simulink model "ds_adc_system"  (R2021b)
settings: Solver=VariableStepAuto  StartTime=0.0  StopTime=1 - 1/5.12e6  RelTol=1e-3
undefined symbols (not defined in the file): a1, a2, b1, b2, c1, c2, DiscIntNeverNeededParam, f, vin
libraries: simulink_extras x2, dspsigops x1
settings Model: Creator=Raymond.Yang  LastModifiedBy=Raymond.Yang
settings SolverCC: AlgebraicLoopSolver=TrustRegion
settings DebuggingCC: SFMachineParentedDataDiag=warning

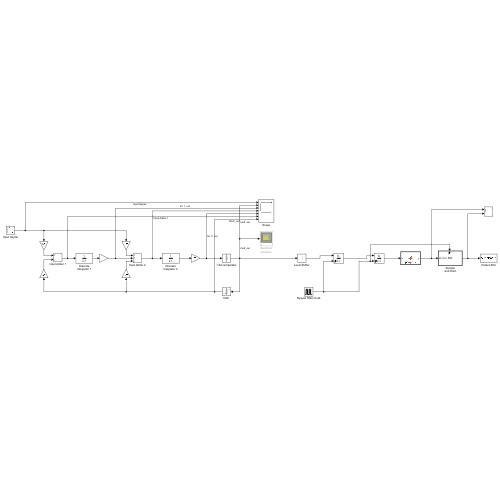
[thumbnail: Simulink's stored preview of the top-level diagram]
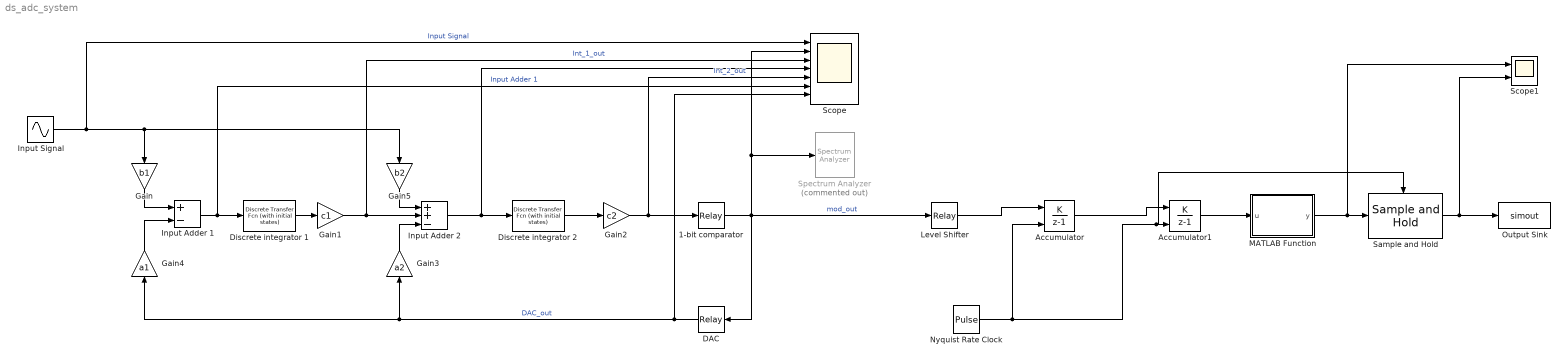
== system ds_adc_system ==
  1-bit comparator : Relay  OnSwitchValue=0  OffSwitchValue=0  OffOutputValue=-1
  Accumulator : DiscreteIntegrator  IntegratorMethod=Accumulation: Forward Euler  ExternalReset=rising  SampleTime=-1  ICPrevOutput=DiscIntNeverNeededParam  ICPrevScaledInput=DiscIntNeverNeededParam
  Accumulator1 : DiscreteIntegrator  IntegratorMethod=Accumulation: Forward Euler  ExternalReset=rising  SampleTime=-1  ICPrevOutput=DiscIntNeverNeededParam  ICPrevScaledInput=DiscIntNeverNeededParam
  DAC : Relay  OnSwitchValue=1  OffSwitchValue=-1  OnOutputValue=0.9  OffOutputValue=-0.9
  Discrete integrator 1 : simulink_extras/Additional Discrete/Discrete Transfer Fcn (with initial states)  N=[1]  D="[1  -1]"  X0=0  TS=-1
      settings: SourceProductBaseCode=SL
  Discrete integrator 2 : simulink_extras/Additional Discrete/Discrete Transfer Fcn (with initial states)  N=[1]  D="[1  -1]"  X0=0  TS=-1
      settings: SourceProductBaseCode=SL
  Gain : Gain  Gain=b1
  Gain1 : Gain  Gain=c1
  Gain2 : Gain  Gain=c2
  Gain3 : Gain  Gain=a2
  Gain4 : Gain  Gain=a1
  Gain5 : Gain  Gain=b2
  Input Adder 1 : Sum  Inputs=+-
  "Input Adder 2 " : Sum  Inputs=++-
  Input Signal : Sin  Amplitude=vin  Frequency=f*2*pi  SampleTime=1/5.12e6
  Level Shifter : Relay  OnSwitchValue=1  OffSwitchValue=-1
  MATLAB Function : MATLAB Function  TreatAsAtomicUnit=on
  Nyquist Rate Clock : DiscretePulseGenerator  PulseType=Time based  Period=1/10e3  PulseWidth=50
  Output Sink : ToWorkspace  VariableName=simout  SaveFormat=Timeseries  SampleTime=-1
  Sample and Hold : dspsigops/Sample and Hold  trig=Rising edge  initCond=0  latchinput=on
  Scope : Scope  NumInputPorts=7
  Scope1 : Scope  NumInputPorts=2
  Spectrum Analyzer : SpectrumAnalyzer  Commented=on
  wires:
  DAC/1 -> Scope/7, Gain4/1, Gain3/1  "DAC_out"
  1-bit comparator/1 -> Level Shifter/1, DAC/1, Scope/2, Spectrum Analyzer/1  "mod_out"
  Input Adder 1/1 -> Scope/6, Discrete integrator 1/1  "Input Adder 1"
  Discrete integrator 1/1 -> Gain1/1
  Input Signal/1 -> Gain/1, Gain5/1, Scope/1  "Input Signal"
  Gain/1 -> Input Adder 1/1
  Gain1/1 -> "Input Adder 2 "/2, Scope/3  "Int_1_out"
  Discrete integrator 2/1 -> Gain2/1
  Gain3/1 -> "Input Adder 2 "/3
  Gain4/1 -> Input Adder 1/2
  "Input Adder 2 "/1 -> Discrete integrator 2/1, Scope/4
  Gain2/1 -> 1-bit comparator/1, Scope/5  "Int_2_out"
  Gain5/1 -> "Input Adder 2 "/1
  Level Shifter/1 -> Accumulator/1
  Accumulator/1 -> Accumulator1/1
  Accumulator1/1 -> MATLAB Function/1(u)
  Nyquist Rate Clock/1 -> Accumulator/2, Sample and Hold/Trigger, Accumulator1/2
  Sample and Hold/1 -> Scope1/2, Output Sink/1
  MATLAB Function/1(y) -> Scope1/1, Sample and Hold/1

== matlab function ds_adc_system/MATLAB Function ==
  data: u input; y output
function y = postproc(u)

    y_17 = mod(u,2);
    u = floor(u/2);
    y_16 = mod(u,2);
    u = floor(u/2);
    y_15 = mod(u,2);
    u = floor(u/2);
    y_14 = mod(u,2);
    u = floor(u/2);
    y_13 = mod(u,2);
    u = floor(u/2);
    y_12 = mod(u,2);
    u = floor(u/2);
    y_11 = mod(u,2);
    u = floor(u/2);
    y_10 = mod(u,2);
    u = floor(u/2);
    y_9 = mod(u,2);
    u = floor(u/2);
    y_8 = mod(u,2);
    u = floor(u/2);
    y_7 = mod(u,2);
    u = floor(u/2);
    y_6 = mod(u,2);
    u = floor(u/2);
    y_5 = mod(u,2);
    u = floor(u/2);
    y_4 = mod(u,2);
    u = floor(u/2);
    y_3 = mod(u,2);
    u = floor(u/2);
    y_2 = mod(u,2);
    u = floor(u/2);
    y_1 = mod(u,2);
    u = floor(u/2);
    y_0 = mod(u,2);

    y = y_11 + y_10*2 + y_9*2^2 + y_8*2^3 + y_7*2^4 + y_6*2^5 + y_5*2^6 + y_4*2^7 + y_3*2^8 + y_2*2^9 + y_1*2^10 + y_0*2^11;

end
